simulink model "discrete_system"  (R2017b)
settings: Solver=ode45  StartTime=0.0  StopTime=10.0  RelTol=1e-3  EnableMultiTasking=on
settings Model: Creator=eechris  LastModifiedBy=eechris
settings DataIOCC: LimitDataPoints=on  SaveFormat=Array  InspectSignalLogs=on
settings OptimizationCC: ExpressionDepthLimit=2147483647  LifeSpan=inf
settings DebuggingCC: UnderspecifiedInitializationDetection=Classic  MergeDetectMultiDrivingBlocksExec=none  SolverPrmCheckMsg=warning  StateNameClashWarn=warning  SFUnexpectedBacktrackingDiag=warning  SFNoUnconditionalDefaultTransitionDiag=warning  SFExecutionAtInitializationDiag=none
settings HardwareCC: ProdBitPerPointer=32  ProdBitPerSizeT=32  ProdBitPerPtrDiffT=32  ProdLargestAtomicFloat=None  ProdIntDivRoundTo=Undefined  ProdEndianess=Unspecified  ProdWordSize=32  ProdHWDeviceType=32-bit Generic
settings ModelReferenceCC: PropagateSignalLabelsOutOfModel=off
settings CodeAppCC: StateflowObjectComments=on
settings GRTTargetCC: TargetLangStandard=C89/C90 (ANSI)  GeneratePreprocessorConditionals=Disable all
settings ConfigComp: CovMetricSettings=dw  CovHtmlReporting=on  CovSaveCumulativeToWorkspaceVar=on  CovSaveSingleToWorkspaceVar=on  CovExternalEMLEnable=off

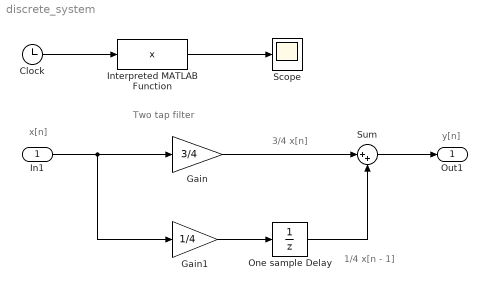
== system discrete_system ==
  note: 1/4 x[n - 1]
  note: 3/4 x[n]
  note: Two tap filter
  note: y[n]
  note: x[n]
  In1 : Inport
  Clock : Clock
  Gain : Gain  Gain=3/4
  Gain1 : Gain  Gain=1/4
  Interpreted MATLAB Function : MATLABFcn  MATLABFcn=x  OutputSignalType=real
  One sample Delay : UnitDelay  SampleTime=-1
  Scope : Scope
  Sum : Sum  Inputs=|++
  Out1 : Outport
  wires:
  Gain1/1 -> One sample Delay/1
  Sum/1 -> Out1/1
  One sample Delay/1 -> Sum/2
  Gain/1 -> Sum/1
  In1/1 -> Gain1/1, Gain/1
  Clock/1 -> Interpreted MATLAB Function/1
  Interpreted MATLAB Function/1 -> Scope/1
